simulink model "valve"  (R2012b)
settings: Solver=ode23t  StartTime=0.0  StopTime=5  RelTol=1e-5
libraries: fl_lib x19, nesl_utility x6, simulink x1
settings Model: Creator=cetaylor  LastModifiedBy=cetaylor

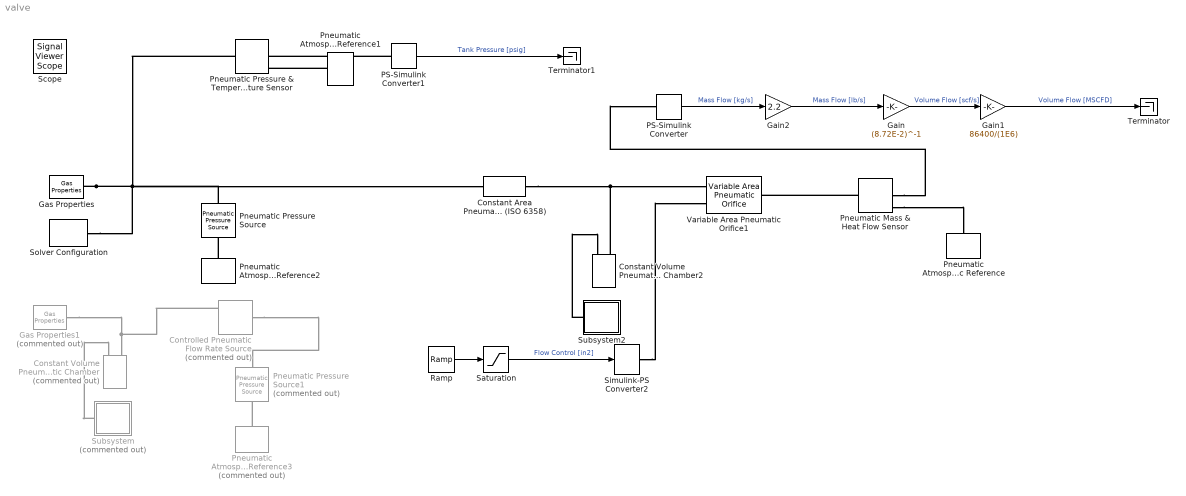
== system valve ==
  Constant Area Pneumatic Orifice (ISO 6358) : fl_lib/Pneumatic/Pneumatic Elements/Constant Area Pneumatic Orifice (ISO 6358)  or_spec=2  sonic_cond=1.6 l/s/bar  area_eff=40/64 in^2  C_v=0.6  K_v=8.5  crit_pr_ratio=0.528  pr_ratio_lam=0.999  T_0=293.15 K  rho_0=1.185 kg/m^3  G_Log=off  Q1_Log=off  Q2_Log=off  p1_Log=off  p2_Log=off  T1_Log=off  T2_Log=off  LocalVarNames=|G|Q1|Q2|p1|p2|T1|T2  LocalVarDescs=|G|Q1|Q2|p1|p2|T1|T2  LocalVarLogging=[0 0 0 0 0 0 0]
  Constant Volume Pneumatic Chamber : fl_lib/Pneumatic/Pneumatic Elements/Constant Volume Pneumatic Chamber  Commented=on  Volume=1500 ft^3  p0=5000 psi  T0=293.15 K  gas_flow_Log=off  heat_flow_Log=off  pressure_Log=off  temperature_Log=off  gas_temperature_Log=off  heat_exch_flow_Log=off  LocalVarNames=|gas_flow|heat_flow|pressure|temperature|gas_temperature|heat_exch_flow  LocalVarDescs=|gas_flow|heat_flow|pressure|temperature|gas_temperature|heat_exch_flow  LocalVarLogging=[0 0 0 0 0 0]
  Constant Volume Pneumatic Chamber2 : fl_lib/Pneumatic/Pneumatic Elements/Constant Volume Pneumatic Chamber  Volume=10 in^3  p0=5000 psi  T0=293.15 K  gas_flow_Log=off  heat_flow_Log=off  pressure_Log=off  temperature_Log=off  gas_temperature_Log=off  heat_exch_flow_Log=off  LocalVarNames=|gas_flow|heat_flow|pressure|temperature|gas_temperature|heat_exch_flow  LocalVarDescs=|gas_flow|heat_flow|pressure|temperature|gas_temperature|heat_exch_flow  LocalVarLogging=[0 0 0 0 0 0]
  Controlled Pneumatic Flow Rate Source : fl_lib/Pneumatic/Pneumatic Sources/Controlled Pneumatic Flow Rate Source  Commented=on  pressure_difference_Log=off  gas_flow_Log=off  temperature_difference_Log=off  heat_flow_Log=off  LocalVarNames=|pressure_difference|gas_flow|temperature_difference|heat_flow  LocalVarDescs=|pressure_difference|gas_flow|temperature_difference|heat_flow  LocalVarLogging=[0 0 0 0]
  Gain : Gain  Gain=(8.72E-2)^-1
  Gain1 : Gain  Gain=86400/(1E6)
  Gain2 : Gain  Gain=2.2
  Gas Properties : fl_lib/Pneumatic/Pneumatic Utilities/Gas Properties  c_p=1005 J/kg/K  c_v=717.95 J/kg/K  viscosity=18.21e-6 s*Pa  Pa=101325 Pa  Ta=293.15 K  LocalVarLogging=[]
  Gas Properties1 : fl_lib/Pneumatic/Pneumatic Utilities/Gas Properties  Commented=on  c_p=1005 J/kg/K  c_v=717.95 J/kg/K  viscosity=18.21e-6 s*Pa  Pa=101325 Pa  Ta=293.15 K  LocalVarLogging=[]
  PS-Simulink Converter : nesl_utility/PS-Simulink Converter  PhysicalDomain=network_engine_domain  LeftPortType=input  RightPortType=output  SubClassName=ps_output  PseudoPeriodic=off  Frequencies=[]  Unit=kg/s  AffineConversion=off
  PS-Simulink Converter1 : nesl_utility/PS-Simulink Converter  PhysicalDomain=network_engine_domain  LeftPortType=input  RightPortType=output  SubClassName=ps_output  PseudoPeriodic=off  Frequencies=[]  Unit=psi  AffineConversion=off
  Pneumatic Atmospheric Reference : fl_lib/Pneumatic/Pneumatic Elements/Pneumatic Atmospheric Reference  gas_flow_Log=off  heat_flow_Log=off  LocalVarNames=|gas_flow|heat_flow  LocalVarDescs=|gas_flow|heat_flow  LocalVarLogging=[0 0]
  Pneumatic Atmospheric Reference1 : fl_lib/Pneumatic/Pneumatic Elements/Pneumatic Atmospheric Reference  gas_flow_Log=off  heat_flow_Log=off  LocalVarNames=|gas_flow|heat_flow  LocalVarDescs=|gas_flow|heat_flow  LocalVarLogging=[0 0]
  Pneumatic Atmospheric Reference2 : fl_lib/Pneumatic/Pneumatic Elements/Pneumatic Atmospheric Reference  gas_flow_Log=off  heat_flow_Log=off  LocalVarNames=|gas_flow|heat_flow  LocalVarDescs=|gas_flow|heat_flow  LocalVarLogging=[0 0]
  Pneumatic Atmospheric Reference3 : fl_lib/Pneumatic/Pneumatic Elements/Pneumatic Atmospheric Reference  Commented=on  gas_flow_Log=off  heat_flow_Log=off  LocalVarNames=|gas_flow|heat_flow  LocalVarDescs=|gas_flow|heat_flow  LocalVarLogging=[0 0]
  Pneumatic Mass & Heat Flow Sensor : fl_lib/Pneumatic/Pneumatic Sensors/Pneumatic Mass & Heat Flow Sensor  pressure_difference_Log=off  gas_flow_Log=off  temperature_difference_Log=off  heat_flow_Log=off  LocalVarNames=|pressure_difference|gas_flow|temperature_difference|heat_flow  LocalVarDescs=|pressure_difference|gas_flow|temperature_difference|heat_flow  LocalVarLogging=[0 0 0 0]
  Pneumatic Pressure & Temperature Sensor : fl_lib/Pneumatic/Pneumatic Sensors/Pneumatic Pressure & Temperature Sensor  pressure_difference_Log=off  gas_flow_Log=off  temperature_difference_Log=off  heat_flow_Log=off  LocalVarNames=|pressure_difference|gas_flow|temperature_difference|heat_flow  LocalVarDescs=|pressure_difference|gas_flow|temperature_difference|heat_flow  LocalVarLogging=[0 0 0 0]
  Pneumatic Pressure Source : fl_lib/Pneumatic/Pneumatic Sources/Pneumatic Pressure Source  pressure_difference_reference=4500 psi  pressure_difference_Log=off  gas_flow_Log=off  temperature_difference_Log=off  heat_flow_Log=off  LocalVarNames=|pressure_difference|gas_flow|temperature_difference|heat_flow  LocalVarDescs=|pressure_difference|gas_flow|temperature_difference|heat_flow  LocalVarLogging=[0 0 0 0]
  Pneumatic Pressure Source1 : fl_lib/Pneumatic/Pneumatic Sources/Pneumatic Pressure Source  Commented=on  pressure_difference_reference=4500 psi  pressure_difference_Log=off  gas_flow_Log=off  temperature_difference_Log=off  heat_flow_Log=off  LocalVarNames=|pressure_difference|gas_flow|temperature_difference|heat_flow  LocalVarDescs=|pressure_difference|gas_flow|temperature_difference|heat_flow  LocalVarLogging=[0 0 0 0]
  Ramp : simulink/Sources/Ramp  slope=.5  start=.1  X0=0
  Saturation : Saturate  UpperLimit=3.14  LowerLimit=0
  Simulink-PS Converter2 : nesl_utility/Simulink-PS Converter  PhysicalDomain=network_engine_domain  LeftPortType=input  RightPortType=output  SubClassName=ps_input  PseudoPeriodic=off  Frequencies=[]  NoiseDistribution=none  NoiseParameters=[]  Unit=in^2  AffineConversion=off  InputFilterTimeConstant=.001  UdotUserProvided=1  SimscapeFilterOrder=1  InputFiltering=off
  Solver Configuration : nesl_utility/Solver Configuration  PhysicalDomain=network_engine_domain  LeftPortType=input  RightPortType=generic  SubClassName=solver  Accelerate=off  Profile=off  UseLocalSampling=off  FrequencyDomain=off  Tones=[]  Harmonics=[]  UseCCode=off  SimulateNoise=off  EnableSwitchedLinearOptims=on  DoDC=on  ResidualTolerance=1e-9  UseLocalSolver=off  LocalSolverChoice=NE_BACKWARD_EULER_ADVANCER  LocalSolverSampleTime=.001  DoFixedCost=off  MaxNonlinIter=3  MaxModeIter=2  LinearAlgebra=Sparse  DelaysMemoryBudget=1024
  Subsystem : Subsystem  Commented=on
  Subsystem2 : Subsystem
  Terminator : Terminator
  Terminator1 : Terminator
  Variable Area Pneumatic Orifice1 : fl_lib/Pneumatic/Pneumatic Elements/Variable Area Pneumatic Orifice  Cd=0.82  Area0=1E-20 in^2  G_Log=off  Q1_Log=off  Q2_Log=off  p1_Log=off  p2_Log=off  T1_Log=off  T2_Log=off  LocalVarNames=|G|Q1|Q2|p1|p2|T1|T2  LocalVarDescs=|G|Q1|Q2|p1|p2|T1|T2  LocalVarLogging=[0 0 0 0 0 0 0]
  Scope : SignalViewerScope  IOType=viewer  NumInputPorts=3  RefreshTime=0.035000
      settings: ShowLegends=on  TimeRange=5  YMin=4275~0~-5  YMax=4725~2.75e-10~5
  wires:
  PS-Simulink Converter/1 -> Gain2/1  "Mass Flow [kg/s]"
  PS-Simulink Converter1/1 -> Terminator1/1  "Tank Pressure [psig]"
  Ramp/1 -> Saturation/1
  Saturation/1 -> Simulink-PS Converter2/1  "Flow Control [in2]"
  Gain/1 -> Gain1/1  "Volume Flow [scf/s]"
  Gain1/1 -> Terminator/1  "Volume Flow [MSCFD]"
  Gain2/1 -> Gain/1  "Mass Flow [lb/s]"
  connections:
  PS-Simulink Converter1/LConn1 -- Pneumatic Pressure & Temperature Sensor/RConn2
  Pneumatic Mass & Heat Flow Sensor/RConn2 -- PS-Simulink Converter/LConn1
  Simulink-PS Converter2/RConn1 -- Variable Area Pneumatic Orifice1/LConn2
  Pneumatic Mass & Heat Flow Sensor/RConn1 -- Pneumatic Atmospheric Reference/LConn1
  Pneumatic Mass & Heat Flow Sensor/LConn1 -- Variable Area Pneumatic Orifice1/RConn1
  Pneumatic Atmospheric Reference1/LConn1 -- Pneumatic Pressure & Temperature Sensor/RConn1
  Constant Volume Pneumatic Chamber2/LConn1 -- Constant Area Pneumatic Orifice (ISO 6358)/RConn1 -- Variable Area Pneumatic Orifice1/LConn1
  Subsystem2/LConn1 -- Constant Volume Pneumatic Chamber2/LConn2
  Subsystem/LConn1 -- Constant Volume Pneumatic Chamber/LConn2
  Gas Properties1/RConn1 -- Controlled Pneumatic Flow Rate Source/RConn1 -- Constant Volume Pneumatic Chamber/LConn1
  Pneumatic Atmospheric Reference2/LConn1 -- Pneumatic Pressure Source/RConn1
  Pneumatic Atmospheric Reference3/LConn1 -- Pneumatic Pressure Source1/RConn1
  Gas Properties/RConn1 -- Constant Area Pneumatic Orifice (ISO 6358)/LConn1 -- Pneumatic Pressure Source/LConn1 -- Solver Configuration/RConn1 -- Pneumatic Pressure & Temperature Sensor/LConn1
  Controlled Pneumatic Flow Rate Source/LConn1 -- Pneumatic Pressure Source1/LConn1

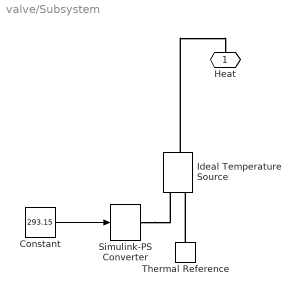
== system valve/Subsystem ==
  Constant : Constant  Value=293.15
  Ideal Temperature Source : fl_lib/Thermal/Thermal Sources/Ideal Temperature Source  Q_Log=off  T_Log=off  LocalVarNames=|Q|T  LocalVarDescs=|Q|T  LocalVarLogging=[0 0]
  Simulink-PS Converter : nesl_utility/Simulink-PS Converter  PhysicalDomain=network_engine_domain  LeftPortType=input  RightPortType=output  SubClassName=ps_input  PseudoPeriodic=off  Frequencies=[]  NoiseDistribution=none  NoiseParameters=[]  Unit=K  AffineConversion=off  InputFilterTimeConstant=.001  UdotUserProvided=1  SimscapeFilterOrder=1  InputFiltering=off
  Thermal Reference : fl_lib/Thermal/Thermal Elements/Thermal Reference  Q_Log=off  LocalVarNames=|Q  LocalVarDescs=|Q  LocalVarLogging=0
  Heat : PMIOPort  Port=1  Side=Left
  wires:
  Constant/1 -> Simulink-PS Converter/1
  connections:
  Ideal Temperature Source/LConn1 -- Heat/RConn1
  Thermal Reference/LConn1 -- Ideal Temperature Source/RConn2
  Simulink-PS Converter/RConn1 -- Ideal Temperature Source/RConn1

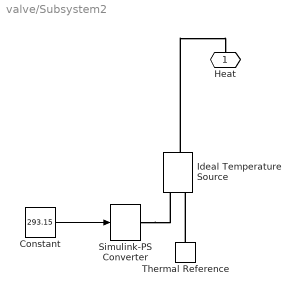
== system valve/Subsystem2 ==
  Constant : Constant  Value=293.15
  Ideal Temperature Source : fl_lib/Thermal/Thermal Sources/Ideal Temperature Source  Q_Log=off  T_Log=off  LocalVarNames=|Q|T  LocalVarDescs=|Q|T  LocalVarLogging=[0 0]
  Simulink-PS Converter : nesl_utility/Simulink-PS Converter  PhysicalDomain=network_engine_domain  LeftPortType=input  RightPortType=output  SubClassName=ps_input  PseudoPeriodic=off  Frequencies=[]  NoiseDistribution=none  NoiseParameters=[]  Unit=K  AffineConversion=off  InputFilterTimeConstant=.001  UdotUserProvided=1  SimscapeFilterOrder=1  InputFiltering=off
  Thermal Reference : fl_lib/Thermal/Thermal Elements/Thermal Reference  Q_Log=off  LocalVarNames=|Q  LocalVarDescs=|Q  LocalVarLogging=0
  Heat : PMIOPort  Port=1  Side=Left
  wires:
  Constant/1 -> Simulink-PS Converter/1
  connections:
  Ideal Temperature Source/LConn1 -- Heat/RConn1
  Thermal Reference/LConn1 -- Ideal Temperature Source/RConn2
  Simulink-PS Converter/RConn1 -- Ideal Temperature Source/RConn1
